simulink model "draft7dot1"  (R2023a)
settings: Solver=VariableStepAuto  StartTime=0.0  StopTime=10  FixedStep=0.0001  MaxStep=0.1  RelTol=1e-3  AbsTol=1e-3  EnableMultiTasking=on
model workspace (MAT data in the model file):
  C_Gimbal = 0.1
  C_IAP = 0.01
  C_Segmental = 0
  IAP_Pa = 0
  K_Gimbal = 0
  K_IAP = 10
  LeftAbdominalMuscleForce = 0
  LeftBackMuscleForce = 0
  LeftTransverse1MuscleForce = 0
  LeftTransverse2MuscleForce = 0
  Moment_AR = 0
  Moment_FE = 7.5
  Moment_LB = 0
  RightAbdominalMuscleForce = 0
  RightBackMuscleForce = 0
  RightTransverse1MuscleForce = 0
  RightTransverse2MuscleForce = 0
  alpha = 1
  beta = 0.7
undefined symbols (not defined in the file or in its folder): X, Y, Z
libraries: sm_lib x269, nesl_utility x215, simulink_extras x33, simulink x15, checkpacklib x3
(part 7 of 7)

== system draft7dot1/L2/AR torque feedback L4 ==
  Constant : Constant  Value=beta
  Constant1 : Constant  Value=C_Segmental
  Discrete Derivative : simulink/Discrete/Discrete Derivative  gainval=1.0  ICPrevScaledInput=0.0  OutMin=[]  OutMax=[]  OutDataType=fixdt(1, 16)  OutScaling=2^-10  DoSatur=off
  Gain5 : Gain  Gain=-1
  PS-Simulink Converter9 : nesl_utility/PS-Simulink Converter  PhysicalDomain=network_engine_domain  SubClassName=ps_output  LeftPortType=input  RightPortType=output  PseudoPeriodic=off  Frequencies=[]  VectorFormat=1-D array  Unit=inherit  AffineConversion=off
  Radians to Degrees : simulink_extras/Transformations/Radians to Degrees
  Simulink-PS Converter6 : nesl_utility/Simulink-PS Converter  PhysicalDomain=network_engine_domain  SubClassName=ps_input  LeftPortType=input  RightPortType=output  PseudoPeriodic=off  Frequencies=[]  NoiseDistribution=none  NoiseParameters=[]  Unit=1  AffineConversion=off  FilteringAndDerivatives=provide  SimscapeFilterOrder=1  InputFilterTimeConstant=0.001  UdotUserProvided=0
  peacewise torque profile5 : MATLAB Function  TreatAsAtomicUnit=on
  AR rot : PMIOPort  Side=Left
  AR torque : PMIOPort  Port=2  Side=Right
  wires:
  Gain5/1 -> Simulink-PS Converter6/1
  peacewise torque profile5/1(torque) -> Gain5/1
  PS-Simulink Converter9/1 -> Radians to Degrees/1
  Radians to Degrees/1 -> Discrete Derivative/1, peacewise torque profile5/1(u)
  Discrete Derivative/1 -> peacewise torque profile5/2(udot)
  Constant/1 -> peacewise torque profile5/3(alpha)
  Constant1/1 -> peacewise torque profile5/4(c)
  connections:
  AR torque/RConn1 -- Simulink-PS Converter6/RConn1
  PS-Simulink Converter9/LConn1 -- AR rot/RConn1

== system draft7dot1/L2/FE torque feedback L4 ==
  Constant : Constant  Value=alpha
  Constant1 : Constant  Value=C_Segmental
  Discrete Derivative : simulink/Discrete/Discrete Derivative  gainval=1.0  ICPrevScaledInput=0.0  OutMin=[]  OutMax=[]  OutDataType=fixdt(1, 16)  OutScaling=2^-10  DoSatur=off
  Gain1 : Gain  Gain=-1
  Gain7 : Gain
  PS-Simulink Converter5 : nesl_utility/PS-Simulink Converter  PhysicalDomain=network_engine_domain  SubClassName=ps_output  LeftPortType=input  RightPortType=output  PseudoPeriodic=off  Frequencies=[]  VectorFormat=1-D array  Unit=inherit  AffineConversion=off
  Radians to Degrees : simulink_extras/Transformations/Radians to Degrees
  Simulink-PS Converter4 : nesl_utility/Simulink-PS Converter  PhysicalDomain=network_engine_domain  SubClassName=ps_input  LeftPortType=input  RightPortType=output  PseudoPeriodic=off  Frequencies=[]  NoiseDistribution=none  NoiseParameters=[]  Unit=1  AffineConversion=off  FilteringAndDerivatives=provide  SimscapeFilterOrder=1  InputFilterTimeConstant=0.001  UdotUserProvided=0
  peacewise torque profile1 : MATLAB Function  TreatAsAtomicUnit=on
  FE rot : PMIOPort  Side=Left
  FE torque : PMIOPort  Port=2  Side=Right
  wires:
  Gain7/1 -> Simulink-PS Converter4/1
  peacewise torque profile1/1(torque) -> Gain7/1
  Radians to Degrees/1 -> Gain1/1
  PS-Simulink Converter5/1 -> Radians to Degrees/1
  Gain1/1 -> Discrete Derivative/1, peacewise torque profile1/1(u)
  Discrete Derivative/1 -> peacewise torque profile1/2(udot)
  Constant/1 -> peacewise torque profile1/3(alpha)
  Constant1/1 -> peacewise torque profile1/4(c)
  connections:
  FE torque/RConn1 -- Simulink-PS Converter4/RConn1
  FE rot/RConn1 -- PS-Simulink Converter5/LConn1

== system draft7dot1/L2/LB torque feedback L4 ==
  Constant : Constant  Value=alpha
  Constant1 : Constant  Value=C_Segmental
  Discrete Derivative : simulink/Discrete/Discrete Derivative  gainval=1.0  ICPrevScaledInput=0.0  OutMin=[]  OutMax=[]  OutDataType=fixdt(1, 16)  OutScaling=2^-10  DoSatur=off
  Gain4 : Gain  Gain=-1
  PS-Simulink Converter8 : nesl_utility/PS-Simulink Converter  PhysicalDomain=network_engine_domain  SubClassName=ps_output  LeftPortType=input  RightPortType=output  PseudoPeriodic=off  Frequencies=[]  VectorFormat=1-D array  Unit=inherit  AffineConversion=off
  Radians to Degrees : simulink_extras/Transformations/Radians to Degrees
  Simulink-PS Converter5 : nesl_utility/Simulink-PS Converter  PhysicalDomain=network_engine_domain  SubClassName=ps_input  LeftPortType=input  RightPortType=output  PseudoPeriodic=off  Frequencies=[]  NoiseDistribution=none  NoiseParameters=[]  Unit=1  AffineConversion=off  FilteringAndDerivatives=provide  SimscapeFilterOrder=1  InputFilterTimeConstant=0.001  UdotUserProvided=0
  peacewise torque profile4 : MATLAB Function  TreatAsAtomicUnit=on
  LB rot : PMIOPort  Side=Left
  LB torque : PMIOPort  Port=2  Side=Right
  wires:
  peacewise torque profile4/1(torque) -> Gain4/1
  PS-Simulink Converter8/1 -> Radians to Degrees/1
  Gain4/1 -> Simulink-PS Converter5/1
  Radians to Degrees/1 -> Discrete Derivative/1, peacewise torque profile4/1(u)
  Discrete Derivative/1 -> peacewise torque profile4/2(udot)
  Constant/1 -> peacewise torque profile4/3(alpha)
  Constant1/1 -> peacewise torque profile4/4(c)
  connections:
  LB rot/RConn1 -- PS-Simulink Converter8/LConn1
  Simulink-PS Converter5/RConn1 -- LB torque/RConn1

== system draft7dot1/L3/AR torque feedback L4 ==
  Constant : Constant  Value=beta
  Constant1 : Constant  Value=C_Segmental
  Discrete Derivative : simulink/Discrete/Discrete Derivative  gainval=1.0  ICPrevScaledInput=0.0  OutMin=[]  OutMax=[]  OutDataType=fixdt(1, 16)  OutScaling=2^-10  DoSatur=off
  Gain5 : Gain  Gain=-1
  PS-Simulink Converter9 : nesl_utility/PS-Simulink Converter  PhysicalDomain=network_engine_domain  SubClassName=ps_output  LeftPortType=input  RightPortType=output  PseudoPeriodic=off  Frequencies=[]  VectorFormat=1-D array  Unit=inherit  AffineConversion=off
  Radians to Degrees : simulink_extras/Transformations/Radians to Degrees
  Simulink-PS Converter6 : nesl_utility/Simulink-PS Converter  PhysicalDomain=network_engine_domain  SubClassName=ps_input  LeftPortType=input  RightPortType=output  PseudoPeriodic=off  Frequencies=[]  NoiseDistribution=none  NoiseParameters=[]  Unit=1  AffineConversion=off  FilteringAndDerivatives=provide  SimscapeFilterOrder=1  InputFilterTimeConstant=0.001  UdotUserProvided=0
  peacewise torque profile5 : MATLAB Function  TreatAsAtomicUnit=on
  AR rot : PMIOPort  Side=Left
  AR torque : PMIOPort  Port=2  Side=Right
  wires:
  peacewise torque profile5/1(torque) -> Gain5/1
  Gain5/1 -> Simulink-PS Converter6/1
  PS-Simulink Converter9/1 -> Radians to Degrees/1
  Radians to Degrees/1 -> Discrete Derivative/1, peacewise torque profile5/1(u)
  Constant/1 -> peacewise torque profile5/3(alpha)
  Constant1/1 -> peacewise torque profile5/4(c)
  Discrete Derivative/1 -> peacewise torque profile5/2(udot)
  connections:
  PS-Simulink Converter9/LConn1 -- AR rot/RConn1
  AR torque/RConn1 -- Simulink-PS Converter6/RConn1

== system draft7dot1/L3/FE torque feedback L4 ==
  Constant : Constant  Value=alpha
  Constant1 : Constant  Value=C_Segmental
  Discrete Derivative : simulink/Discrete/Discrete Derivative  gainval=1.0  ICPrevScaledInput=0.0  OutMin=[]  OutMax=[]  OutDataType=fixdt(1, 16)  OutScaling=2^-10  DoSatur=off
  Gain1 : Gain  Gain=-1
  Gain7 : Gain
  PS-Simulink Converter5 : nesl_utility/PS-Simulink Converter  PhysicalDomain=network_engine_domain  SubClassName=ps_output  LeftPortType=input  RightPortType=output  PseudoPeriodic=off  Frequencies=[]  VectorFormat=1-D array  Unit=inherit  AffineConversion=off
  Radians to Degrees : simulink_extras/Transformations/Radians to Degrees
  Simulink-PS Converter4 : nesl_utility/Simulink-PS Converter  PhysicalDomain=network_engine_domain  SubClassName=ps_input  LeftPortType=input  RightPortType=output  PseudoPeriodic=off  Frequencies=[]  NoiseDistribution=none  NoiseParameters=[]  Unit=1  AffineConversion=off  FilteringAndDerivatives=provide  SimscapeFilterOrder=1  InputFilterTimeConstant=0.001  UdotUserProvided=0
  peacewise torque profile1 : MATLAB Function  TreatAsAtomicUnit=on
  FE rot : PMIOPort  Side=Left
  FE torque : PMIOPort  Port=2  Side=Right
  wires:
  peacewise torque profile1/1(torque) -> Gain7/1
  Gain7/1 -> Simulink-PS Converter4/1
  Radians to Degrees/1 -> Gain1/1
  PS-Simulink Converter5/1 -> Radians to Degrees/1
  Gain1/1 -> Discrete Derivative/1, peacewise torque profile1/1(u)
  Constant/1 -> peacewise torque profile1/3(alpha)
  Constant1/1 -> peacewise torque profile1/4(c)
  Discrete Derivative/1 -> peacewise torque profile1/2(udot)
  connections:
  FE rot/RConn1 -- PS-Simulink Converter5/LConn1
  FE torque/RConn1 -- Simulink-PS Converter4/RConn1

== system draft7dot1/L3/LB torque feedback L4 ==
  Constant : Constant  Value=alpha
  Constant1 : Constant  Value=C_Segmental
  Discrete Derivative : simulink/Discrete/Discrete Derivative  gainval=1.0  ICPrevScaledInput=0.0  OutMin=[]  OutMax=[]  OutDataType=fixdt(1, 16)  OutScaling=2^-10  DoSatur=off
  Gain4 : Gain  Gain=-1
  PS-Simulink Converter8 : nesl_utility/PS-Simulink Converter  PhysicalDomain=network_engine_domain  SubClassName=ps_output  LeftPortType=input  RightPortType=output  PseudoPeriodic=off  Frequencies=[]  VectorFormat=1-D array  Unit=inherit  AffineConversion=off
  Radians to Degrees : simulink_extras/Transformations/Radians to Degrees
  Simulink-PS Converter5 : nesl_utility/Simulink-PS Converter  PhysicalDomain=network_engine_domain  SubClassName=ps_input  LeftPortType=input  RightPortType=output  PseudoPeriodic=off  Frequencies=[]  NoiseDistribution=none  NoiseParameters=[]  Unit=1  AffineConversion=off  FilteringAndDerivatives=provide  SimscapeFilterOrder=1  InputFilterTimeConstant=0.001  UdotUserProvided=0
  peacewise torque profile4 : MATLAB Function  TreatAsAtomicUnit=on
  LB rot : PMIOPort  Side=Left
  LB torque : PMIOPort  Port=2  Side=Right
  wires:
  Gain4/1 -> Simulink-PS Converter5/1
  PS-Simulink Converter8/1 -> Radians to Degrees/1
  peacewise torque profile4/1(torque) -> Gain4/1
  Radians to Degrees/1 -> Discrete Derivative/1, peacewise torque profile4/1(u)
  Discrete Derivative/1 -> peacewise torque profile4/2(udot)
  Constant/1 -> peacewise torque profile4/3(alpha)
  Constant1/1 -> peacewise torque profile4/4(c)
  connections:
  Simulink-PS Converter5/RConn1 -- LB torque/RConn1
  LB rot/RConn1 -- PS-Simulink Converter8/LConn1

== system draft7dot1/L4/AR torque feedback L4 ==
  Constant : Constant  Value=beta
  Constant1 : Constant  Value=C_Segmental
  Discrete Derivative : simulink/Discrete/Discrete Derivative  gainval=1.0  ICPrevScaledInput=0.0  OutMin=[]  OutMax=[]  OutDataType=fixdt(1, 16)  OutScaling=2^-10  DoSatur=off
  Gain5 : Gain  Gain=-1
  PS-Simulink Converter9 : nesl_utility/PS-Simulink Converter  PhysicalDomain=network_engine_domain  SubClassName=ps_output  LeftPortType=input  RightPortType=output  PseudoPeriodic=off  Frequencies=[]  VectorFormat=1-D array  Unit=inherit  AffineConversion=off
  Radians to Degrees : simulink_extras/Transformations/Radians to Degrees
  Simulink-PS Converter6 : nesl_utility/Simulink-PS Converter  PhysicalDomain=network_engine_domain  SubClassName=ps_input  LeftPortType=input  RightPortType=output  PseudoPeriodic=off  Frequencies=[]  NoiseDistribution=none  NoiseParameters=[]  Unit=1  AffineConversion=off  FilteringAndDerivatives=provide  SimscapeFilterOrder=1  InputFilterTimeConstant=0.001  UdotUserProvided=0
  peacewise torque profile5 : MATLAB Function  TreatAsAtomicUnit=on
  AR rot : PMIOPort  Side=Left
  AR torque : PMIOPort  Port=2  Side=Right
  wires:
  Gain5/1 -> Simulink-PS Converter6/1
  peacewise torque profile5/1(torque) -> Gain5/1
  PS-Simulink Converter9/1 -> Radians to Degrees/1
  Radians to Degrees/1 -> Discrete Derivative/1, peacewise torque profile5/1(u)
  Constant/1 -> peacewise torque profile5/3(alpha)
  Constant1/1 -> peacewise torque profile5/4(c)
  Discrete Derivative/1 -> peacewise torque profile5/2(udot)
  connections:
  AR torque/RConn1 -- Simulink-PS Converter6/RConn1
  PS-Simulink Converter9/LConn1 -- AR rot/RConn1

== system draft7dot1/L4/FE torque feedback L4 ==
  Constant : Constant  Value=alpha
  Constant1 : Constant  Value=C_Segmental
  Discrete Derivative : simulink/Discrete/Discrete Derivative  gainval=1.0  ICPrevScaledInput=0.0  OutMin=[]  OutMax=[]  OutDataType=fixdt(1, 16)  OutScaling=2^-10  DoSatur=off
  Gain1 : Gain  Gain=-1
  Gain7 : Gain
  PS-Simulink Converter5 : nesl_utility/PS-Simulink Converter  PhysicalDomain=network_engine_domain  SubClassName=ps_output  LeftPortType=input  RightPortType=output  PseudoPeriodic=off  Frequencies=[]  VectorFormat=1-D array  Unit=inherit  AffineConversion=off
  Radians to Degrees : simulink_extras/Transformations/Radians to Degrees
  Simulink-PS Converter4 : nesl_utility/Simulink-PS Converter  PhysicalDomain=network_engine_domain  SubClassName=ps_input  LeftPortType=input  RightPortType=output  PseudoPeriodic=off  Frequencies=[]  NoiseDistribution=none  NoiseParameters=[]  Unit=1  AffineConversion=off  FilteringAndDerivatives=provide  SimscapeFilterOrder=1  InputFilterTimeConstant=0.001  UdotUserProvided=0
  peacewise torque profile1 : MATLAB Function  TreatAsAtomicUnit=on
  FE rot : PMIOPort  Side=Left
  FE torque : PMIOPort  Port=2  Side=Right
  wires:
  Gain7/1 -> Simulink-PS Converter4/1
  peacewise torque profile1/1(torque) -> Gain7/1
  Radians to Degrees/1 -> Gain1/1
  PS-Simulink Converter5/1 -> Radians to Degrees/1
  Gain1/1 -> Discrete Derivative/1, peacewise torque profile1/1(u)
  Discrete Derivative/1 -> peacewise torque profile1/2(udot)
  Constant/1 -> peacewise torque profile1/3(alpha)
  Constant1/1 -> peacewise torque profile1/4(c)
  connections:
  FE torque/RConn1 -- Simulink-PS Converter4/RConn1
  FE rot/RConn1 -- PS-Simulink Converter5/LConn1

== system draft7dot1/L4/LB torque feedback L4 ==
  Constant : Constant  Value=alpha
  Constant1 : Constant  Value=C_Segmental
  Discrete Derivative : simulink/Discrete/Discrete Derivative  gainval=1.0  ICPrevScaledInput=0.0  OutMin=[]  OutMax=[]  OutDataType=fixdt(1, 16)  OutScaling=2^-10  DoSatur=off
  Gain4 : Gain  Gain=-1
  PS-Simulink Converter8 : nesl_utility/PS-Simulink Converter  PhysicalDomain=network_engine_domain  SubClassName=ps_output  LeftPortType=input  RightPortType=output  PseudoPeriodic=off  Frequencies=[]  VectorFormat=1-D array  Unit=inherit  AffineConversion=off
  Radians to Degrees : simulink_extras/Transformations/Radians to Degrees
  Simulink-PS Converter5 : nesl_utility/Simulink-PS Converter  PhysicalDomain=network_engine_domain  SubClassName=ps_input  LeftPortType=input  RightPortType=output  PseudoPeriodic=off  Frequencies=[]  NoiseDistribution=none  NoiseParameters=[]  Unit=1  AffineConversion=off  FilteringAndDerivatives=provide  SimscapeFilterOrder=1  InputFilterTimeConstant=0.001  UdotUserProvided=0
  peacewise torque profile4 : MATLAB Function  TreatAsAtomicUnit=on
  LB rot : PMIOPort  Side=Left
  LB torque : PMIOPort  Port=2  Side=Right
  wires:
  peacewise torque profile4/1(torque) -> Gain4/1
  PS-Simulink Converter8/1 -> Radians to Degrees/1
  Gain4/1 -> Simulink-PS Converter5/1
  Radians to Degrees/1 -> Discrete Derivative/1, peacewise torque profile4/1(u)
  Constant/1 -> peacewise torque profile4/3(alpha)
  Constant1/1 -> peacewise torque profile4/4(c)
  Discrete Derivative/1 -> peacewise torque profile4/2(udot)
  connections:
  LB rot/RConn1 -- PS-Simulink Converter8/LConn1
  Simulink-PS Converter5/RConn1 -- LB torque/RConn1

== system draft7dot1/L5/AR torque feedback L5 ==
  Constant : Constant  Value=beta
  Constant1 : Constant  Value=C_Segmental
  Discrete Derivative : simulink/Discrete/Discrete Derivative  gainval=1.0  ICPrevScaledInput=0.0  OutMin=[]  OutMax=[]  OutDataType=fixdt(1, 16)  OutScaling=2^-10  DoSatur=off
  Gain2 : Gain  Gain=-1
  PS-Simulink Converter3 : nesl_utility/PS-Simulink Converter  PhysicalDomain=network_engine_domain  SubClassName=ps_output  LeftPortType=input  RightPortType=output  PseudoPeriodic=off  Frequencies=[]  VectorFormat=1-D array  Unit=inherit  AffineConversion=off
  Radians to Degrees : simulink_extras/Transformations/Radians to Degrees
  Simulink-PS Converter2 : nesl_utility/Simulink-PS Converter  PhysicalDomain=network_engine_domain  SubClassName=ps_input  LeftPortType=input  RightPortType=output  PseudoPeriodic=off  Frequencies=[]  NoiseDistribution=none  NoiseParameters=[]  Unit=1  AffineConversion=off  FilteringAndDerivatives=provide  SimscapeFilterOrder=1  InputFilterTimeConstant=0.001  UdotUserProvided=0
  peacewise torque profile3 : MATLAB Function  TreatAsAtomicUnit=on
  AR rot : PMIOPort  Side=Left
  AR torque : PMIOPort  Port=2  Side=Right
  wires:
  peacewise torque profile3/1(torque) -> Gain2/1
  Gain2/1 -> Simulink-PS Converter2/1
  PS-Simulink Converter3/1 -> Radians to Degrees/1
  Radians to Degrees/1 -> Discrete Derivative/1, peacewise torque profile3/1(u)
  Constant/1 -> peacewise torque profile3/3(alpha)
  Constant1/1 -> peacewise torque profile3/4(c)
  Discrete Derivative/1 -> peacewise torque profile3/2(udot)
  connections:
  AR torque/RConn1 -- Simulink-PS Converter2/RConn1
  PS-Simulink Converter3/LConn1 -- AR rot/RConn1

== system draft7dot1/L5/FE torque feedback L5 ==
  Constant : Constant  Value=alpha
  Constant1 : Constant  Value=C_Segmental
  Discrete Derivative : simulink/Discrete/Discrete Derivative  gainval=1.0  ICPrevScaledInput=0.0  OutMin=[]  OutMax=[]  OutDataType=fixdt(1, 16)  OutScaling=2^-10  DoSatur=off
  Gain1 : Gain  Gain=-1
  Gain6 : Gain
  PS-Simulink Converter : nesl_utility/PS-Simulink Converter  PhysicalDomain=network_engine_domain  SubClassName=ps_output  LeftPortType=input  RightPortType=output  PseudoPeriodic=off  Frequencies=[]  VectorFormat=inherit  Unit=inherit  AffineConversion=off
  Radians to Degrees : simulink_extras/Transformations/Radians to Degrees
  Simulink-PS Converter3 : nesl_utility/Simulink-PS Converter  PhysicalDomain=network_engine_domain  SubClassName=ps_input  LeftPortType=input  RightPortType=output  PseudoPeriodic=off  Frequencies=[]  NoiseDistribution=none  NoiseParameters=[]  Unit=1  AffineConversion=off  FilteringAndDerivatives=provide  SimscapeFilterOrder=1  InputFilterTimeConstant=0.001  UdotUserProvided=0
  peacewise torque profile (+- 15 deg) : MATLAB Function  TreatAsAtomicUnit=on
  FE torque : PMIOPort  Side=Right
  FE rot : PMIOPort  Port=2  Side=Left
  wires:
  Gain6/1 -> Simulink-PS Converter3/1  "moment"
  peacewise torque profile (+- 15 deg)/1(torque) -> Gain6/1
  Radians to Degrees/1 -> Gain1/1
  PS-Simulink Converter/1 -> Radians to Degrees/1
  Gain1/1 -> Discrete Derivative/1, peacewise torque profile (+- 15 deg)/1(u)  "rot"
  Discrete Derivative/1 -> peacewise torque profile (+- 15 deg)/2(udot)
  Constant/1 -> peacewise torque profile (+- 15 deg)/3(alpha)
  Constant1/1 -> peacewise torque profile (+- 15 deg)/4(c)
  connections:
  FE rot/RConn1 -- PS-Simulink Converter/LConn1
  Simulink-PS Converter3/RConn1 -- FE torque/RConn1

== system draft7dot1/L5/LB torque feedback L5 ==
  Constant : Constant  Value=alpha
  Constant1 : Constant  Value=C_Segmental
  Discrete Derivative : simulink/Discrete/Discrete Derivative  gainval=1.0  ICPrevScaledInput=0.0  OutMin=[]  OutMax=[]  OutDataType=fixdt(1, 16)  OutScaling=2^-10  DoSatur=off
  Gain1 : Gain  Gain=-1
  PS-Simulink Converter2 : nesl_utility/PS-Simulink Converter  PhysicalDomain=network_engine_domain  SubClassName=ps_output  LeftPortType=input  RightPortType=output  PseudoPeriodic=off  Frequencies=[]  VectorFormat=1-D array  Unit=inherit  AffineConversion=off
  Radians to Degrees : simulink_extras/Transformations/Radians to Degrees
  Simulink-PS Converter1 : nesl_utility/Simulink-PS Converter  PhysicalDomain=network_engine_domain  SubClassName=ps_input  LeftPortType=input  RightPortType=output  PseudoPeriodic=off  Frequencies=[]  NoiseDistribution=none  NoiseParameters=[]  Unit=1  AffineConversion=off  FilteringAndDerivatives=provide  SimscapeFilterOrder=1  InputFilterTimeConstant=0.001  UdotUserProvided=0
  peacewise torque profile2 : MATLAB Function  TreatAsAtomicUnit=on
  LB rot : PMIOPort  Side=Left
  LB torque : PMIOPort  Port=2  Side=Right
  wires:
  Gain1/1 -> Simulink-PS Converter1/1
  PS-Simulink Converter2/1 -> Radians to Degrees/1
  peacewise torque profile2/1(torque) -> Gain1/1
  Radians to Degrees/1 -> Discrete Derivative/1, peacewise torque profile2/1(u)
  Discrete Derivative/1 -> peacewise torque profile2/2(udot)
  Constant/1 -> peacewise torque profile2/3(alpha)
  Constant1/1 -> peacewise torque profile2/4(c)
  connections:
  LB rot/RConn1 -- PS-Simulink Converter2/LConn1
  Simulink-PS Converter1/RConn1 -- LB torque/RConn1

== matlab function draft7dot1/L2/AR torque feedback L4/peacewise torque profile5 ==
  data: u input; torque output; udot input; alpha input; c input
% function torque = T(u,a,b)    % Panjabi data fitted into logarithmic equation. Refer validation.xlsx
%     torque = 0;
%     if (u >= 0)
%      torque= a*(exp(u/0.80)-1)/0.93;
% 
%     elseif (u < 0)
%      torque= b*(exp(u/-2.72)-1)/(-0.10)   ;
% end

function torque = T(u,udot,alpha,c)    % Panjabi data fitted into logarithmic equation. Refer validation.xlsx
    torque = 0;
    if (u >= 0)
     torque= alpha* ( (exp(u/0.80)-1)/0.93  +  c*udot  );

    elseif (u < 0)
     torque= alpha* ( (exp(u/-2.72)-1)/(-0.10)   +  c*udot  ) ;
end

== matlab function draft7dot1/L2/FE torque feedback L4/peacewise torque profile1 ==
  data: u input; torque output; udot input; alpha input; c input
function torque = T(u,udot,alpha,c) 
    torque = 0;
    if (u >= 0)
     torque= alpha* ( (exp(u/8.23)-1)/0.10 +  c*udot  )  ;

    elseif (u< 0)
     torque= alpha* ( (exp(u/-1.31)-1)/(-0.58) +  c*udot  )  ;
end





% function torque = T(u,a,b) % Guan et al logarithmic
%     torque = 0;
%     if (u >= 0)
%      torque= a*(exp(u/8.23)-1)/0.10;
% 
%     elseif (u< 0)
%      torque= b*(exp(u/-1.31)-1)/(-0.58)   ;
% end

% function torque = T(u,a,b) % Rao et al segmental
%     torque = 0;
%     if (u >= 0)
%         torque= (a)*(-0.0042*u^2 + 1.9155*u);
%     elseif (u< 0)
%         torque= (b)*(-0.0042*u^2 + 1.9155*u);
% end

== matlab function draft7dot1/L2/LB torque feedback L4/peacewise torque profile4 ==
  data: u input; torque output; udot input; alpha input; c input
function torque = T(u,udot,alpha,c)    % Guan et al (nonlinear logarithmic equation mentioned in their paper)
    torque = 0;
    if (u >= 0)
     torque= alpha* ( (exp(u/2.13)-1)/0.87  +  c*udot  );

    elseif (u< 0)
     torque= alpha* ( (exp(u/-2.22)-1)/(-0.66) + c*udot  )  ;
end

== matlab function draft7dot1/L1/AR torque feedback L4/peacewise torque profile5 ==
  data: u input; torque output; udot input; alpha input; c input
% function torque = T(u,a,b)    % Panjabi data fitted into logarithmic equation. Refer validation.xlsx
%     torque = 0;
%     if (u >= 0)
%      torque= a*(exp(u/0.83)-1)/0.35;
% 
%     elseif (u < 0)
%      torque= b*(exp(u/-0.38)-1)/(-3.18)   ;
% end


function torque = T(u,udot,alpha,c)    
    torque = 0;
    if (u >= 0)
     torque= alpha* ( (exp(u/0.83)-1)/0.35   +  c*udot  );

    elseif (u < 0)
     torque= alpha* (  (exp(u/-0.38)-1)/(-3.18)  +  c*udot  )  ;
end

== matlab function draft7dot1/L1/FE torque feedback L4/peacewise torque profile1 ==
  data: u input; torque output; udot input; alpha input; c input
function torque = T(u,udot,alpha,c)  % Guan et al logarithmic  (RECALCULATED - refer excel)
    torque = 0;
    if (u >= 0)
     torque= alpha* (  (exp(u/8.067)-1)/0.1031  +  c*udot  );

    elseif (u < 0)
     torque= alpha* ( (exp(u/-1.2951)-1)/(-0.5753)   +  c*udot  )  ;
end



% function torque = T(u,a,b)  % Guan et al logarithmic  (RECALCULATED - refer excel)
%     torque = 0;
%     if (u >= 0)
%      torque= a*(exp(u/8.067)-1)/0.1031;
% 
%     elseif (u < 0)
%      torque= b*(exp(u/-1.2951)-1)/(-0.5753)   ;
% end


% function torque = T(u,a,b)  % Rao et al segmental
%     torque = 0;
%     if (u >= 0)
%         torque = (a)*(0.0343*u^2 + 1.9989*u);
%     elseif (u < 0)
%         torque = (b)*(0.0343*u^2 + 1.9989*u);
% end

== matlab function draft7dot1/L4/FE torque feedback L4/peacewise torque profile1 ==
  data: u input; torque output; udot input; alpha input; c input


function torque = T(u,udot,alpha,c) % Guan et al logarithmic
    torque = 0;
    if (u >= 0)
     torque= alpha* ( (exp(u/3.07)-1)/0.81  +  c*udot  );

    elseif (u< 0)
     torque= alpha* ( (exp(u/-8.14)-1)/(-0.05) +  c*udot  )  ;
end

% function torque = T(u,a,b) % Rao et al segmental
%     torque = 0;
%     if (u >= 0)
%         torque= (a)*(0.0493*u^2 + 2.2629*u);
%     elseif (u< 0)
%         torque= (b)*(0.0493*u^2 + 2.2629*u);
% end

== matlab function draft7dot1/L1/LB torque feedback L4/peacewise torque profile4 ==
  data: u input; torque output; udot input; alpha input; c input
% function torque = T(u,a,b)    % Guan et al (RECALCULATED - refer excel)
%     torque = 0;
%     if (u >= 0)
%      torque= a*(exp(u/2.0545)-1)/0.9457;
% 
%     elseif (u< 0)
%      torque= b*(exp(u/-2.3716)-1)/(-0.5744)   ;
% end


function torque = T(u,udot,alpha,c)   
    torque = 0;
    if (u >= 0)
     torque= alpha* ( (exp(u/2.0545)-1)/0.9457   +  c*udot  );

    elseif (u< 0)
     torque= alpha* ( (exp(u/-2.3716)-1)/(-0.5744)  +  c*udot   ) ;
end

== matlab function draft7dot1/Muscle Forces/Sum of Square of Forces ==
  data: F1 input; SumofSquareofForces output; F2 input; F3 input; F4 input; F5 input; F6 input; F7 input; F8 input; IAP input
function SumofSquareofForces = fcn(F1,F2,F3,F4,F5,F6,F7,F8,IAP)

SumofSquareofForces = F1^2 + F2^2 + F3^2 + F4^2 + F5^2 + F6^2 +F7^2 + F8^2 + IAP^2;

== matlab function draft7dot1/L5/FE torque feedback L5/peacewise torque profile (+- 15 deg) ==
  data: u input; torque output; udot input; alpha input; c input


function torque = T(u,udot,alpha,c)    % Guan et al (nonlinear logarithmic equation mentioned in their paper)
    torque = 0;
    if (u >= 0)
     torque= alpha* ( (exp(u/5.58)-1)/0.59  +  c*udot  );

    elseif (u< 0)
     torque= alpha* ( (exp(u/-4.48)-1)/(-0.33) +  c*udot  )  ;
end

% function torque = T(u,a,b)    % Rao et al segmental data
%     torque = 0;
%     if (u >= 0)
%         torque= (a)*(0.0348*u^3 + 0.089*u^2 + 1.1837*u);
%     elseif (u< 0)
%         torque= (b)*(0.0348*u^3 + 0.089*u^2 + 1.1837*u);
% end

== matlab function draft7dot1/L5/LB torque feedback L5/peacewise torque profile2 ==
  data: u input; torque output; udot input; alpha input; c input
function torque = T(u,udot,alpha,c)    % Guan et al (nonlinear logarithmic equation mentioned in their paper)
    torque = 0;
    if (u >= 0)
     torque= alpha* ( (exp(u/3.26)-1)/0.49  +  c*udot  );

    elseif (u < 0)
     torque= alpha* ( (exp(u/-4.22)-1)/(-0.29)  +  c*udot  ) ;
end

== matlab function draft7dot1/L5/AR torque feedback L5/peacewise torque profile3 ==
  data: u input; torque output; udot input; alpha input; c input
function torque = T(u,udot,alpha,c)    % Panjabi data fitted into logarithmic equation. Refer validation.xlsx
    torque = 0;
    if (u >= 0)
     torque= alpha* ( (exp(u/1.25)-1)/0.10  +  c*udot  );

    elseif (u < 0)
     torque= alpha* ( (exp(u/-1.05)-1)/(-0.10)  +  c*udot  )  ;
end

== matlab function draft7dot1/L4/LB torque feedback L4/peacewise torque profile4 ==
  data: u input; torque output; udot input; alpha input; c input
function torque = T(u,udot,alpha,c)    % Guan et al (nonlinear logarithmic equation mentioned in their paper)
    torque = 0;
    if (u >= 0)
     torque= alpha* ( (exp(u/1.77)-1)/1.28  + c*udot  );

    elseif (u< 0)
     torque= alpha* ( (exp(u/-1.44)-1)/(-1.23)  + c*udot  )  ;
end

== matlab function draft7dot1/L4/AR torque feedback L4/peacewise torque profile5 ==
  data: u input; torque output; udot input; alpha input; c input
% function torque = T(u,a,b)    % Panjabi data fitted into logarithmic equation. Refer validation.xlsx
%     torque = 0;
%     if (u >= 0)
%      torque= a*(exp(u/0.73)-1)/0.20;
% 
%     elseif (u < 0)
%      torque= b*(exp(u/-1.01)-1)/(-0.31)   ;
% end



function torque = T(u,udot,alpha,c)    % Panjabi data fitted into logarithmic equation. Refer validation.xlsx
    torque = 0;
    if (u >= 0)
     torque= alpha* (  (exp(u/0.73)-1)/0.20  +  c*udot  ) ;

    elseif (u < 0)
     torque= alpha* ( (exp(u/-1.01)-1)/(-0.31)  +  c*udot  )  ;
end

== matlab function draft7dot1/L3/AR torque feedback L4/peacewise torque profile5 ==
  data: u input; torque output; udot input; alpha input; c input
function torque = T(u,udot,alpha,c)    % Panjabi data fitted into logarithmic equation. Refer validation.xlsx
    torque = 0;
    if (u >= 0)
     torque= alpha* ( (exp(u/2.69)-1)/0.10  +  c*udot  );

    elseif (u < 0)
     torque= alpha* ( (exp(u/-0.90)-1)/(-0.89)  +  c*udot  )  ;
end

== matlab function draft7dot1/L3/FE torque feedback L4/peacewise torque profile1 ==
  data: u input; torque output; udot input; alpha input; c input
function torque = T(u,udot,alpha,c)  % Guan et al logarithmic
    torque = 0;
    if (u >= 0)
     torque= alpha* ( (exp(u/11.09)-1)/0.09  +  c*udot  );

    elseif (u< 0)
     torque= alpha* ( (exp(u/-24.35)-1)/(-0.02)  +  c*udot  ) ;
end


% function torque = T(u,a,b)  % Guan et al logarithmic
%     torque = 0;
%     if (u >= 0)
%      torque= a*(exp(u/11.09)-1)/0.09;
% 
%     elseif (u< 0)
%      torque= b*(exp(u/-24.35)-1)/(-0.02)   ;
% end

% function torque = T(u,a,b)  % Rao et al segmental
%     torque = 0;
%     if (u >= 0)
%         torque = (a)*(0.0342*u^3 + 0.0596*u^2 + 1.5861*u);
%     elseif (u< 0)
%         torque = (b)*(0.0342*u^3 + 0.0596*u^2 + 1.5861*u);
% end

== matlab function draft7dot1/L3/LB torque feedback L4/peacewise torque profile4 ==
  data: u input; torque output; udot input; alpha input; c input
% function torque = T(u,a,b)    % Guan et al (nonlinear logarithmic equation mentioned in their paper)
%     torque = 0;
%     if (u >= 0)
%      torque= a*(exp(u/2.50)-1)/1.02;
% 
%     elseif (u< 0)
%      torque= b*(exp(u/-2.58)-1)/(-0.82)   ;
% end

function torque = T(u,udot,alpha,c)    % Guan et al (nonlinear logarithmic equation mentioned in their paper)
    torque = 0;
    if (u >= 0)
     torque= alpha* ( (exp(u/2.50)-1)/1.02  +  c*udot  );

    elseif (u< 0)
     torque= alpha* ( (exp(u/-2.58)-1)/(-0.82)   +  c*udot )  ;
end
